simulink model "pid_n_wrm"  (R2015a)
settings: Solver=ode45  StartTime=0.0  StopTime=10.0  RelTol=1e-3
libraries: simulink x2
settings Model: Creator=rojas-j  LastModifiedBy=rojas-j

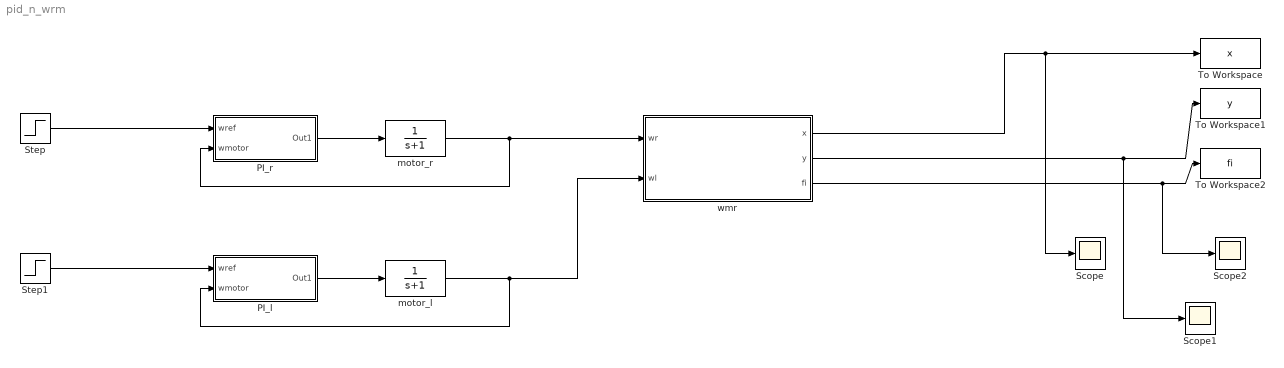
== system pid_n_wrm ==
  PI_l : Subsystem
  PI_r : Subsystem
  Scope : Scope
  Scope1 : Scope
  Scope2 : Scope
      settings: SaveName=ScopeData2
  Step : Step  SampleTime=0
  Step1 : Step  SampleTime=0
  To Workspace : ToWorkspace  VariableName=x  SaveFormat=Timeseries  SampleTime=-1
  To Workspace1 : ToWorkspace  VariableName=y  SaveFormat=Timeseries  SampleTime=-1
  To Workspace2 : ToWorkspace  VariableName=fi  SaveFormat=Timeseries  SampleTime=-1
  motor_l : TransferFcn  Denominator=[1 1]
  motor_r : TransferFcn  Denominator=[1 1]
  wmr : Subsystem
  wires:
  wmr/1(x) -> Scope/1, To Workspace/1
  wmr/2(y) -> Scope1/1, To Workspace1/1
  wmr/3(fi) -> Scope2/1, To Workspace2/1
  PI_r/1(Out1) -> motor_r/1
  motor_r/1 -> PI_r/2(wmotor), wmr/1(wr)
  PI_l/1(Out1) -> motor_l/1
  motor_l/1 -> wmr/2(wl), PI_l/2(wmotor)
  Step/1 -> PI_r/1(wref)
  Step1/1 -> PI_l/1(wref)

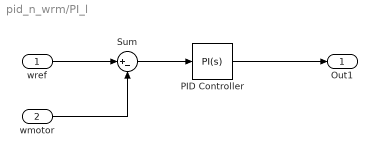
== system pid_n_wrm/PI_l ==
  wref : Inport
  wmotor : Inport  Port=2
  PID Controller : simulink/Continuous/PID Controller  Controller=PI  TimeDomain=Continuous-time  SampleTime=-1  IntegratorMethod=Forward Euler  FilterMethod=Forward Euler  Form=Parallel  UseFilter=on  ControllerParametersSource=internal  P=7  I=16  D=0  N=100  InitialConditionSource=internal  InitialConditionForIntegrator=0  InitialConditionForFilter=0  ExternalReset=none  LimitOutput=off  UpperSaturationLimit=inf  LowerSaturationLimit=-inf  LinearizeAsGain=on  AntiWindupMode=none  Kb=1  TrackingMode=off  Kt=1  PParamMin=[]  PParamMax=[]  IParamMin=[]  IParamMax=[]  DParamMin=[]  DParamMax=[]  NParamMin=[]  NParamMax=[]  KbParamMin=[]  KbParamMax=[]  KtParamMin=[]  KtParamMax=[]  POutMin=[]  POutMax=[]  IOutMin=[]  IOutMax=[]  DOutMin=[]  DOutMax=[]  NOutMin=[]  NOutMax=[]  KbOutMin=[]  KbOutMax=[]  KtOutMin=[]  KtOutMax=[]  IntegratorOutMin=[]  IntegratorOutMax=[]  FilterOutMin=[]  FilterOutMax=[]  SumOutMin=[]  SumOutMax=[]  SumI1OutMin=[]  SumI1OutMax=[]  SumI2OutMin=[]  SumI2OutMax=[]  SumI3OutMin=[]  SumI3OutMax=[]  SumDOutMin=[]  SumDOutMax=[]  SaturationOutMin=[]  SaturationOutMax=[]  IntegratorContinuousStateAttributes=''  IntegratorStateMustResolveToSignalObject=off  IntegratorRTWStateStorageClass=Auto  FilterContinuousStateAttributes=''  FilterStateMustResolveToSignalObject=off  FilterRTWStateStorageClass=Auto  DifferentiatorICPrevScaledInput=0  DifferentiatorOutMin=[]  DifferentiatorOutMax=[]
  Sum : Sum  Inputs=|+-
  Out1 : Outport
  wires:
  Sum/1 -> PID Controller/1
  wref/1 -> Sum/1
  wmotor/1 -> Sum/2
  PID Controller/1 -> Out1/1

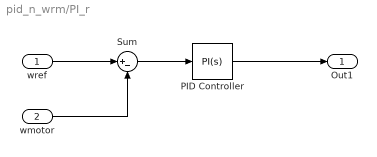
== system pid_n_wrm/PI_r ==
  wref : Inport
  wmotor : Inport  Port=2
  PID Controller : simulink/Continuous/PID Controller  Controller=PI  TimeDomain=Continuous-time  SampleTime=-1  IntegratorMethod=Forward Euler  FilterMethod=Forward Euler  Form=Parallel  UseFilter=on  ControllerParametersSource=internal  P=7  I=16  D=0  N=100  InitialConditionSource=internal  InitialConditionForIntegrator=0  InitialConditionForFilter=0  ExternalReset=none  LimitOutput=off  UpperSaturationLimit=inf  LowerSaturationLimit=-inf  LinearizeAsGain=on  AntiWindupMode=none  Kb=1  TrackingMode=off  Kt=1  PParamMin=[]  PParamMax=[]  IParamMin=[]  IParamMax=[]  DParamMin=[]  DParamMax=[]  NParamMin=[]  NParamMax=[]  KbParamMin=[]  KbParamMax=[]  KtParamMin=[]  KtParamMax=[]  POutMin=[]  POutMax=[]  IOutMin=[]  IOutMax=[]  DOutMin=[]  DOutMax=[]  NOutMin=[]  NOutMax=[]  KbOutMin=[]  KbOutMax=[]  KtOutMin=[]  KtOutMax=[]  IntegratorOutMin=[]  IntegratorOutMax=[]  FilterOutMin=[]  FilterOutMax=[]  SumOutMin=[]  SumOutMax=[]  SumI1OutMin=[]  SumI1OutMax=[]  SumI2OutMin=[]  SumI2OutMax=[]  SumI3OutMin=[]  SumI3OutMax=[]  SumDOutMin=[]  SumDOutMax=[]  SaturationOutMin=[]  SaturationOutMax=[]  IntegratorContinuousStateAttributes=''  IntegratorStateMustResolveToSignalObject=off  IntegratorRTWStateStorageClass=Auto  FilterContinuousStateAttributes=''  FilterStateMustResolveToSignalObject=off  FilterRTWStateStorageClass=Auto  DifferentiatorICPrevScaledInput=0  DifferentiatorOutMin=[]  DifferentiatorOutMax=[]
  Sum : Sum  Inputs=|+-
  Out1 : Outport
  wires:
  Sum/1 -> PID Controller/1
  wref/1 -> Sum/1
  wmotor/1 -> Sum/2
  PID Controller/1 -> Out1/1

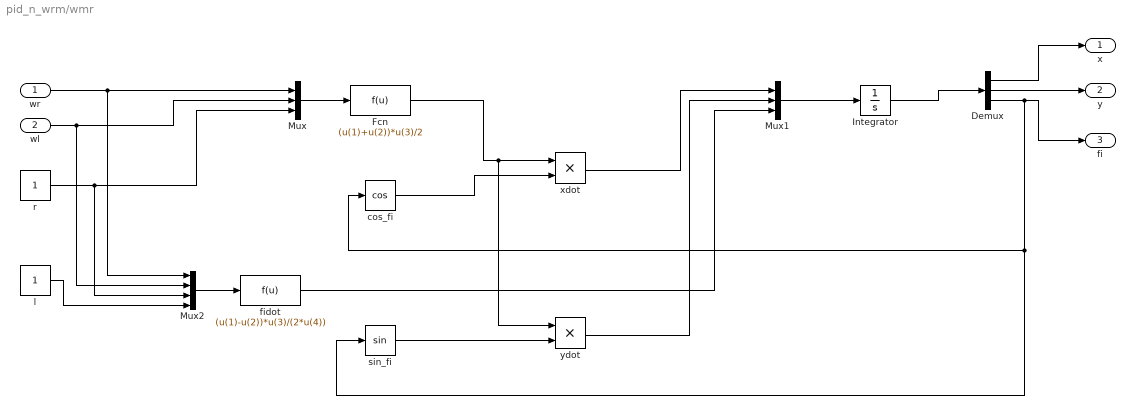
== system pid_n_wrm/wmr ==
  wr : Inport
  wl : Inport  Port=2
  Demux : Demux  Outputs=3
  Fcn : Fcn  Expr=(u(1)+u(2))*u(3)/2
  Integrator : Integrator
  Mux : Mux  Inputs=3
  Mux1 : Mux  Inputs=3
  Mux2 : Mux
  "cos_fi " : Trigonometry  Operator=cos
  fidot : Fcn  Expr=(u(1)-u(2))*u(3)/(2*u(4))
  l : Constant
  r : Constant
  "sin_fi " : Trigonometry
  xdot : Product
  ydot : Product
  x : Outport
  y : Outport  Port=2
  fi : Outport  Port=3
  wires:
  wr/1 -> Mux2/1, Mux/1
  wl/1 -> Mux2/2, Mux/2
  Mux/1 -> Fcn/1
  Mux1/1 -> Integrator/1
  Integrator/1 -> Demux/1
  Demux/1 -> x/1
  Demux/2 -> y/1
  Demux/3 -> "sin_fi "/1, "cos_fi "/1, fi/1
  Fcn/1 -> ydot/1, xdot/1
  "cos_fi "/1 -> xdot/2
  xdot/1 -> Mux1/1
  "sin_fi "/1 -> ydot/2
  r/1 -> Mux2/3, Mux/3
  ydot/1 -> Mux1/2
  Mux2/1 -> fidot/1
  l/1 -> Mux2/4
  fidot/1 -> Mux1/3
